simulink model "DC_2a_th"  (R2022b)
settings: Solver=VariableStepAuto  StartTime=0.0  StopTime=tEnd  MaxStep=1e-5  RelTol=1e-3
values from neighbouring files (symbols this model uses):
  C1 = 4e-6    (= 4e-06)    [DC_2_th.m]
  L1 = 10e-3    (= 0.01)    [DC_2_th.m]
  R1 = 68    [DC_2_th.m]
settings Model: Creator=alici  LastModifiedBy=alici

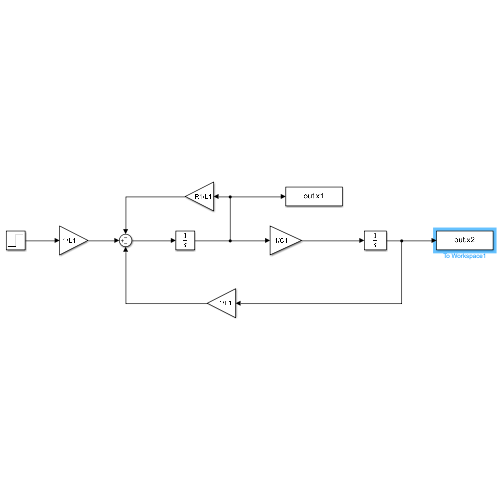
[thumbnail: Simulink's stored preview of the top-level diagram]
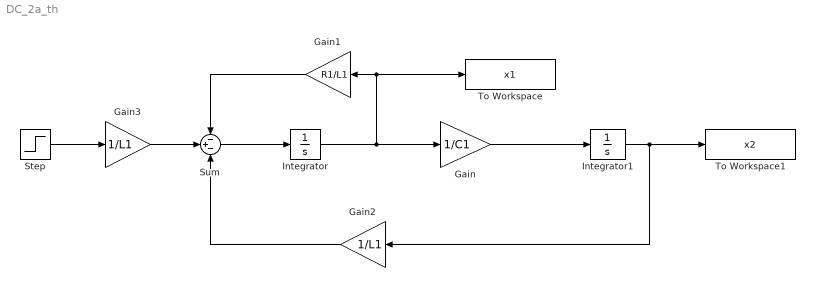
== system DC_2a_th ==
  Gain : Gain  Gain=1/C1
  Gain1 : Gain  Gain=R1/L1
  Gain2 : Gain  Gain=1/L1
  Gain3 : Gain  Gain=1/L1
  Integrator : Integrator
  Integrator1 : Integrator
  Step : Step  Time=0  SampleTime=0
  Sum : Sum  Inputs=-+-
  To Workspace : ToWorkspace  VariableName=x1  SaveFormat=Timeseries  SampleTime=-1
  To Workspace1 : ToWorkspace  VariableName=x2  SaveFormat=Timeseries  SampleTime=-1
  wires:
  Integrator/1 -> To Workspace/1, Gain1/1, Gain/1
  Gain/1 -> Integrator1/1
  Sum/1 -> Integrator/1
  Gain1/1 -> Sum/1
  Integrator1/1 -> To Workspace1/1, Gain2/1
  Gain2/1 -> Sum/3
  Step/1 -> Gain3/1
  Gain3/1 -> Sum/2
